simulink model "axis_controller"  (R2020a)
settings: Solver=VariableStepAuto  StartTime=0.0  StopTime=inf  RelTol=1e-3
InitFcn:
  | f_system = 256e6;
libraries: hdlsllib x2
settings Model: Creator=david  LastModifiedBy=david
settings OptimizationCC: BlockReduction=off  ConditionallyExecuteInputs=off  DefaultParameterBehavior=Inlined
settings DebuggingCC: AlgebraicLoopMsg=error
settings HardwareCC: ProdBitPerPointer=32  ProdBitPerSizeT=32  ProdBitPerPtrDiffT=32  ProdLargestAtomicFloat=None  ProdIntDivRoundTo=Undefined  ProdEndianess=Unspecified  ProdWordSize=32  ProdHWDeviceType=ASIC/FPGA->ASIC/FPGA  TargetBitPerPointer=64  TargetBitPerSizeT=64  TargetBitPerPtrDiffT=64  TargetLongLongMode=on  TargetIntDivRoundTo=Zero  TargetEndianess=LittleEndian  TargetWordSize=64  TargetHWDeviceType=Custom Processor->MATLAB Host Computer  ProdEqTarget=off

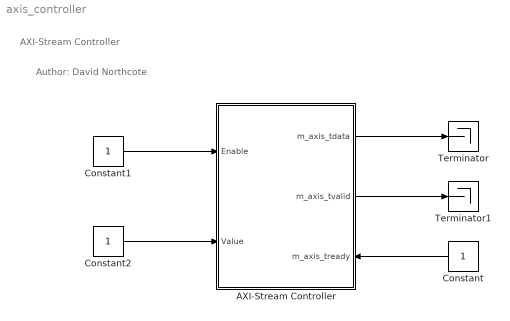
== system axis_controller ==
  note: Author: David Northcote
  note: AXI-Stream Controller
  AXI-Stream Controller : Subsystem  TreatAsAtomicUnit=on
      settings: PortSchema="{\"entries\":[{\"content\":{\"sides\":[{\"content\":{\"connectorIds\":[\"In1\",\"In2\"]},\"type\":\"ConnectorPlacement.EquallySpacedRectSide\",\"uuid\":\"239a9995-0b8c-494e-a673-86dd79e3ecbc\"},{\"content\":{\"connectorIds\":[\"Out1\",\"Out2\",\"In3\"],\"side\":\"RIGHT\"},\"type\":\"ConnectorPlacement.EquallySpacedRectSide\",\"uuid\":\"2e32a57b-a30e-49d7-a7e9-0e4be6c7949e\"},{\"content\":{\"connectorIds\":[],\"side\":\"TOP\"},\"type\":\"ConnectorPlacement.EquallySpacedRectSide\",\"uuid\":\"0fe3c5fd-6b2b-4864-8f33-4697d91e188d\"}]},\"type\":\"ConnectorPlacement.EquallySpacedConnector\",\"uuid\":\"659fe604-1a06-443f-bb23-1784571a6596\"}],\"packageUris\":[\"http://schema.mathworks.com/mf0/Connector/19700101\"],\"version\":\"1.0\"}"
  Constant : Constant  OutDataTypeStr=boolean  SampleTime=-1
  Constant1 : Constant  OutDataTypeStr=uint32  SampleTime=-1
  Constant2 : Constant  OutDataTypeStr=uint32  SampleTime=-1
  Terminator : Terminator
  Terminator1 : Terminator
  wires:
  AXI-Stream Controller/1(m_axis_tdata) -> Terminator/1
  AXI-Stream Controller/2(m_axis_tvalid) -> Terminator1/1
  Constant/1 -> AXI-Stream Controller/3(m_axis_tready)
  Constant1/1 -> AXI-Stream Controller/1(Enable)
  Constant2/1 -> AXI-Stream Controller/2(Value)

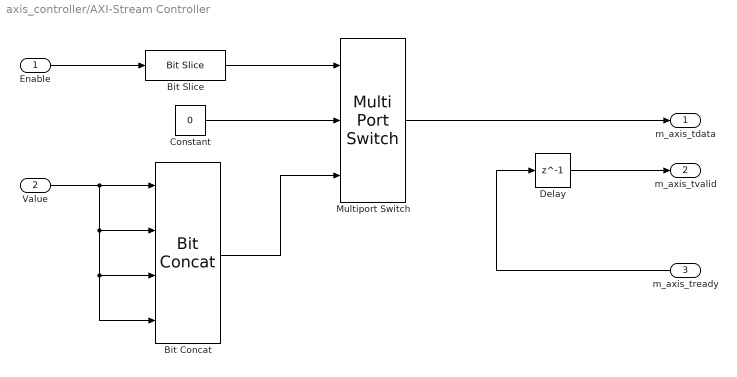
== system axis_controller/AXI-Stream Controller ==
  Enable : Inport
  Value : Inport  Port=2
  m_axis_tready : Inport  Port=3
  Bit Concat : hdlsllib/Logic and Bit Operations/Bit Concat  numInputs=4
  Bit Slice : hdlsllib/Logic and Bit Operations/Bit Slice  lidx=0  ridx=0
      settings: SourceProductBaseCode=SL
  Constant : Constant  Value=0  OutDataTypeStr=Inherit: Inherit via back propagation  SampleTime=-1
  Delay : Delay  DelayLength=1
  Multiport Switch : MultiPortSwitch  DataPortOrder=Zero-based contiguous  Inputs=2  zeroidx=on
  m_axis_tdata : Outport
  m_axis_tvalid : Outport  Port=2
  wires:
  Delay/1 -> m_axis_tvalid/1
  m_axis_tready/1 -> Delay/1
  Bit Slice/1 -> Multiport Switch/1
  Multiport Switch/1 -> m_axis_tdata/1
  Constant/1 -> Multiport Switch/2
  Enable/1 -> Bit Slice/1
  Bit Concat/1 -> Multiport Switch/3
  Value/1 -> Bit Concat/4, Bit Concat/3, Bit Concat/2, Bit Concat/1
